simulink model "sum1"  (R2016b)
settings: Solver=ode3  StartTime=0.0  StopTime=20  FixedStep=0.01  RelTol=1e-3
settings Model: Creator=byalant  LastModifiedBy=byalant

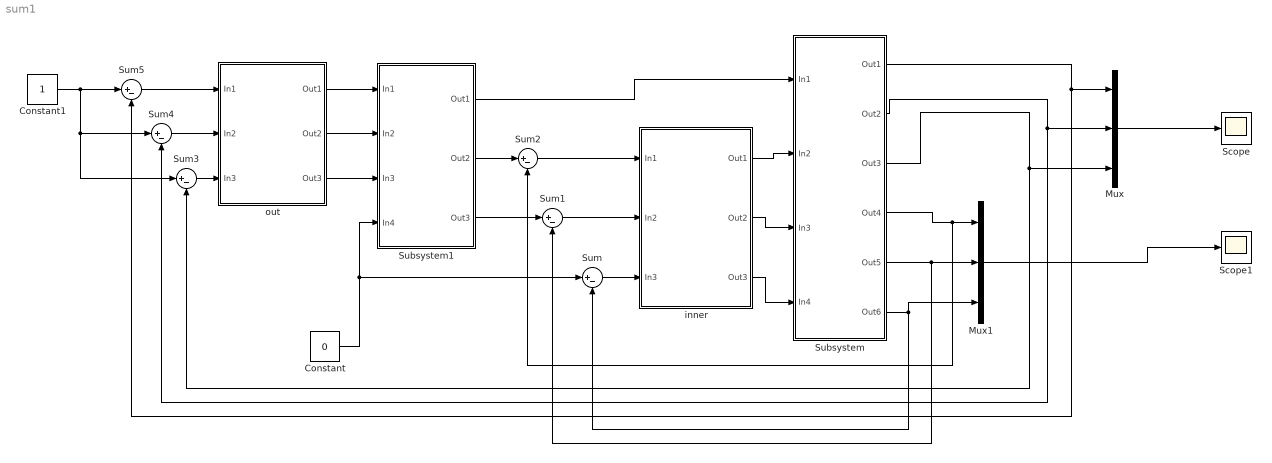
== system sum1 ==
  Constant : Constant  Value=0
  Constant1 : Constant
  Mux : Mux  Inputs=3
  Mux1 : Mux  Inputs=3
  Scope : Scope
  Scope1 : Scope
  Subsystem : Subsystem
  Subsystem1 : Subsystem
  Sum{,1..5} (6 alike) : Sum  Inputs=|+-
  inner : Subsystem
  out : Subsystem
  wires:
  inner/1(Out1) -> Subsystem/2(In2)
  inner/2(Out2) -> Subsystem/3(In3)
  inner/3(Out3) -> Subsystem/4(In4)
  Sum/1 -> inner/3(In3)
  Sum1/1 -> inner/2(In2)
  Sum2/1 -> inner/1(In1)
  out/1(Out1) -> Subsystem1/1(In1)
  out/2(Out2) -> Subsystem1/2(In2)
  out/3(Out3) -> Subsystem1/3(In3)
  Subsystem1/2(Out2) -> Sum2/1
  Subsystem1/3(Out3) -> Sum1/1
  Subsystem1/1(Out1) -> Subsystem/1(In1)
  Constant/1 -> Sum/1, Subsystem1/4(In4)
  Subsystem/2(Out2) -> Sum4/2, Mux/2
  Subsystem/1(Out1) -> Sum5/2, Mux/1
  Subsystem/4(Out4) -> Sum2/2, Mux1/1
  Subsystem/5(Out5) -> Mux1/2, Sum1/2
  Subsystem/6(Out6) -> Mux1/3, Sum/2
  Sum3/1 -> out/3(In3)
  Sum4/1 -> out/2(In2)
  Sum5/1 -> out/1(In1)
  Subsystem/3(Out3) -> Sum3/2, Mux/3
  Mux/1 -> Scope/1
  Constant1/1 -> Sum3/1, Sum4/1, Sum5/1
  Mux1/1 -> Scope1/1

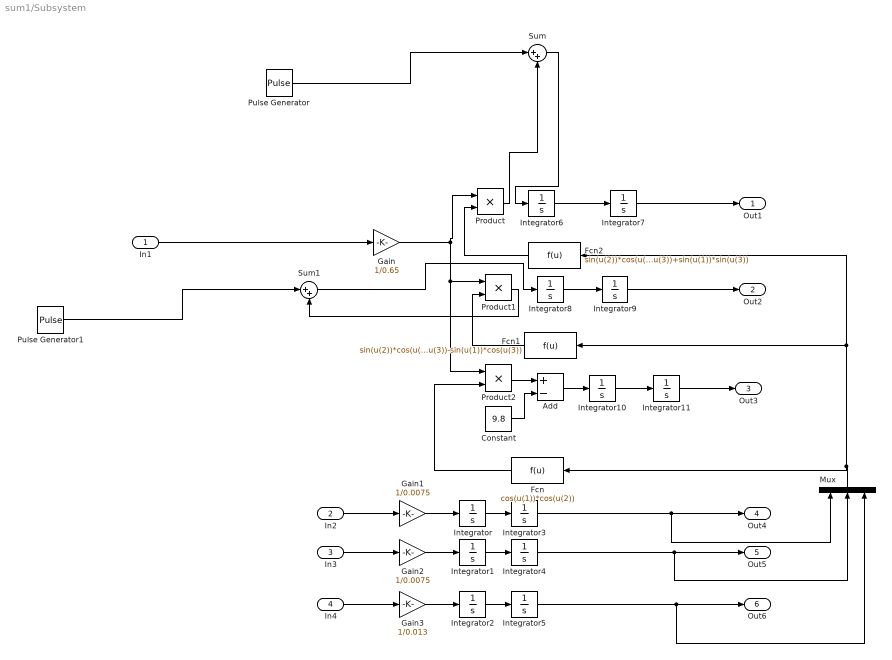
== system sum1/Subsystem ==
  In1 : Inport
  In2 : Inport  Port=2
  In3 : Inport  Port=3
  In4 : Inport  Port=4
  Add : Sum  Inputs=+-
  Constant : Constant  Value=9.8
  Fcn : Fcn  Expr=cos(u(1))*cos(u(2))
  Fcn1 : Fcn  Expr=sin(u(2))*cos(u(1))*sin(u(3))-sin(u(1))*cos(u(3))
  Fcn2 : Fcn  Expr=sin(u(2))*cos(u(1))*cos(u(3))+sin(u(1))*sin(u(3))
  Gain : Gain  Gain=1/0.65
  Gain1 : Gain  Gain=1/0.0075
  Gain2 : Gain  Gain=1/0.0075
  Gain3 : Gain  Gain=1/0.013
  Integrator{,1..11} (12 alike) : Integrator
  Mux : Mux  Inputs=3
  Product : Product
  Product1 : Product
  Product2 : Product
  Pulse Generator : DiscretePulseGenerator  PulseType=Time based  PulseWidth=50
  Pulse Generator1 : DiscretePulseGenerator  PulseType=Time based  PulseWidth=50
  Sum : Sum  Inputs=|++
  Sum1 : Sum  Inputs=|++
  Out1 : Outport
  Out2 : Outport  Port=2
  Out3 : Outport  Port=3
  Out4 : Outport  Port=4
  Out5 : Outport  Port=5
  Out6 : Outport  Port=6
  wires:
  In2/1 -> Gain1/1
  In3/1 -> Gain2/1
  In4/1 -> Gain3/1
  Gain1/1 -> Integrator/1
  Gain2/1 -> Integrator1/1
  Gain3/1 -> Integrator2/1
  Integrator/1 -> Integrator3/1
  Integrator1/1 -> Integrator4/1
  Integrator2/1 -> Integrator5/1
  Integrator6/1 -> Integrator7/1
  Integrator8/1 -> Integrator9/1
  Integrator10/1 -> Integrator11/1
  Integrator11/1 -> Out3/1
  Integrator9/1 -> Out2/1
  Integrator7/1 -> Out1/1
  Fcn/1 -> Product2/2
  Fcn2/1 -> Product/2
  Fcn1/1 -> Product1/2
  Integrator3/1 -> Mux/1, Out4/1
  Integrator4/1 -> Mux/2, Out5/1
  Integrator5/1 -> Out6/1, Mux/3
  Product2/1 -> Add/1
  Constant/1 -> Add/2
  Add/1 -> Integrator10/1
  Gain/1 -> Product/1, Product2/1, Product1/1
  In1/1 -> Gain/1
  Mux/1 -> Fcn2/1, Fcn1/1, Fcn/1
  Pulse Generator/1 -> Sum/1
  Sum/1 -> Integrator6/1
  Product/1 -> Sum/2
  Pulse Generator1/1 -> Sum1/1
  Sum1/1 -> Integrator8/1
  Product1/1 -> Sum1/2

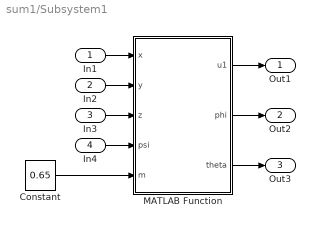
== system sum1/Subsystem1 ==
  In1 : Inport
  In2 : Inport  Port=2
  In3 : Inport  Port=3
  In4 : Inport  Port=4
  Constant : Constant  Value=0.65
  MATLAB Function : MATLAB Function  TreatAsAtomicUnit=on
  Out1 : Outport
  Out2 : Outport  Port=2
  Out3 : Outport  Port=3
  wires:
  In4/1 -> MATLAB Function/4(psi)
  In1/1 -> MATLAB Function/1(x)
  In2/1 -> MATLAB Function/2(y)
  In3/1 -> MATLAB Function/3(z)
  MATLAB Function/1(u1) -> Out1/1
  MATLAB Function/2(phi) -> Out2/1
  MATLAB Function/3(theta) -> Out3/1
  Constant/1 -> MATLAB Function/5(m)

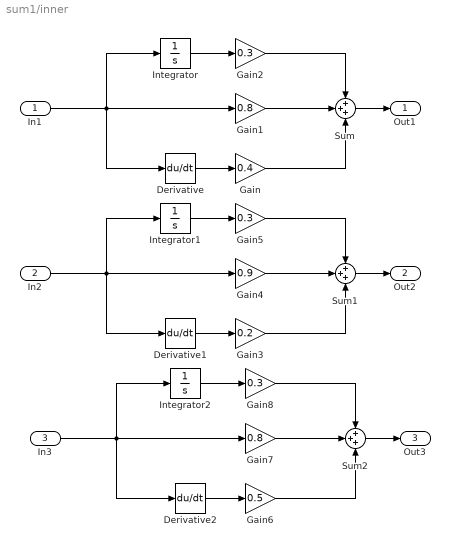
== system sum1/inner ==
  In1 : Inport
  In2 : Inport  Port=2
  In3 : Inport  Port=3
  Derivative : Derivative
  Derivative1 : Derivative
  Derivative2 : Derivative
  Gain : Gain  Gain=0.4
  Gain1 : Gain  Gain=0.8
  Gain2 : Gain  Gain=0.3
  Gain3 : Gain  Gain=0.2
  Gain4 : Gain  Gain=0.9
  Gain5 : Gain  Gain=0.3
  Gain6 : Gain  Gain=0.5
  Gain7 : Gain  Gain=0.8
  Gain8 : Gain  Gain=0.3
  Integrator : Integrator
  Integrator1 : Integrator
  Integrator2 : Integrator
  Sum : Sum  Inputs=+++
  Sum1 : Sum  Inputs=+++
  Sum2 : Sum  Inputs=+++
  Out1 : Outport
  Out2 : Outport  Port=2
  Out3 : Outport  Port=3
  wires:
  Gain1/1 -> Sum/2
  Gain2/1 -> Sum/1
  Gain/1 -> Sum/3
  Integrator/1 -> Gain2/1
  In1/1 -> Derivative/1, Integrator/1, Gain1/1
  Derivative/1 -> Gain/1
  Sum/1 -> Out1/1
  Gain4/1 -> Sum1/2
  Gain5/1 -> Sum1/1
  Gain3/1 -> Sum1/3
  Integrator1/1 -> Gain5/1
  In2/1 -> Derivative1/1, Integrator1/1, Gain4/1
  Derivative1/1 -> Gain3/1
  Sum1/1 -> Out2/1
  Gain7/1 -> Sum2/2
  Gain8/1 -> Sum2/1
  Gain6/1 -> Sum2/3
  Integrator2/1 -> Gain8/1
  In3/1 -> Derivative2/1, Integrator2/1, Gain7/1
  Derivative2/1 -> Gain6/1
  Sum2/1 -> Out3/1

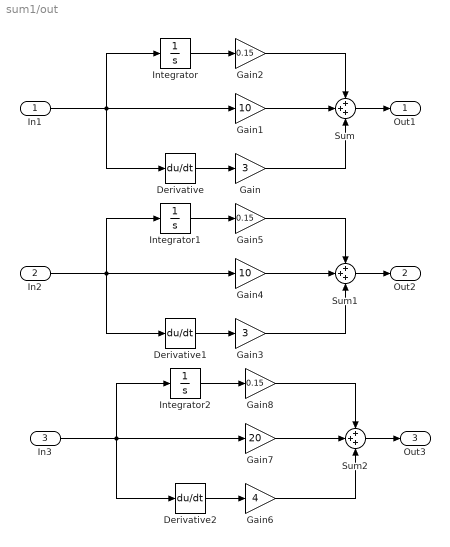
== system sum1/out ==
  In1 : Inport
  In2 : Inport  Port=2
  In3 : Inport  Port=3
  Derivative : Derivative
  Derivative1 : Derivative
  Derivative2 : Derivative
  Gain : Gain  Gain=3
  Gain1 : Gain  Gain=10
  Gain2 : Gain  Gain=0.15
  Gain3 : Gain  Gain=3
  Gain4 : Gain  Gain=10
  Gain5 : Gain  Gain=0.15
  Gain6 : Gain  Gain=4
  Gain7 : Gain  Gain=20
  Gain8 : Gain  Gain=0.15
  Integrator : Integrator
  Integrator1 : Integrator
  Integrator2 : Integrator
  Sum : Sum  Inputs=+++
  Sum1 : Sum  Inputs=+++
  Sum2 : Sum  Inputs=+++
  Out1 : Outport
  Out2 : Outport  Port=2
  Out3 : Outport  Port=3
  wires:
  Gain1/1 -> Sum/2
  Gain2/1 -> Sum/1
  Gain/1 -> Sum/3
  Integrator/1 -> Gain2/1
  In1/1 -> Derivative/1, Integrator/1, Gain1/1
  Derivative/1 -> Gain/1
  Sum/1 -> Out1/1
  Gain4/1 -> Sum1/2
  Gain5/1 -> Sum1/1
  Gain3/1 -> Sum1/3
  Integrator1/1 -> Gain5/1
  In2/1 -> Derivative1/1, Integrator1/1, Gain4/1
  Derivative1/1 -> Gain3/1
  Sum1/1 -> Out2/1
  Gain7/1 -> Sum2/2
  Gain8/1 -> Sum2/1
  Gain6/1 -> Sum2/3
  Integrator2/1 -> Gain8/1
  In3/1 -> Derivative2/1, Integrator2/1, Gain7/1
  Derivative2/1 -> Gain6/1
  Sum2/1 -> Out3/1

== matlab function sum1/Subsystem1/MATLAB Function ==
  data: u1 output; x input; phi output; y input; z input; theta output; psi input; m input
function [u1,phi,theta] = fcn(x,y,z,psi,m)
u1=m*sqrt((x^2+y^2+(z+9.8)^2));
phi=asin(m*(x*sin(psi)-y*cos(psi))/u1);
s=m*(x*sin(psi)-y*cos(psi))/u1;
c=sqrt(1-s*s);

theta=asin((m*x-sin(psi)*s)/(u1*cos(psi)*c));
end
